simulink model "lab3_simulink"  (R2023b)
settings: Solver=VariableStepAuto  StartTime=0.0  StopTime=150  RelTol=1e-3
values from neighbouring files (symbols this model uses):
  G = tf(num, den, 'IOdelay', Tm)    [lab3.m]
  HR = tf(numHR, denHR, Ts)    [lab3.m]
  HR1 = tf(numHR, denHR1, Ts)    [lab3.m]
settings Model: Creator=Voic  LastModifiedBy=Voic
settings OptimizationCC: ReuseModelBlockBuffer=off

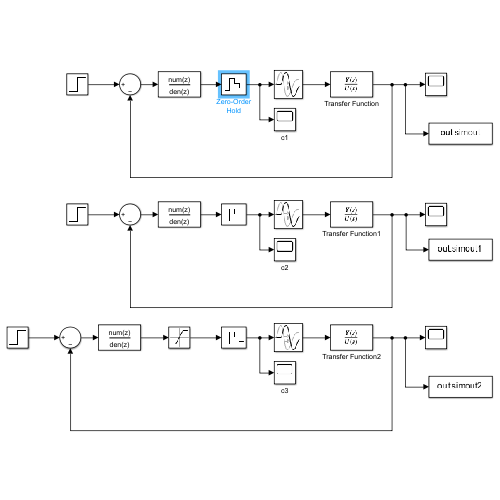
[thumbnail: Simulink's stored preview of the top-level diagram]
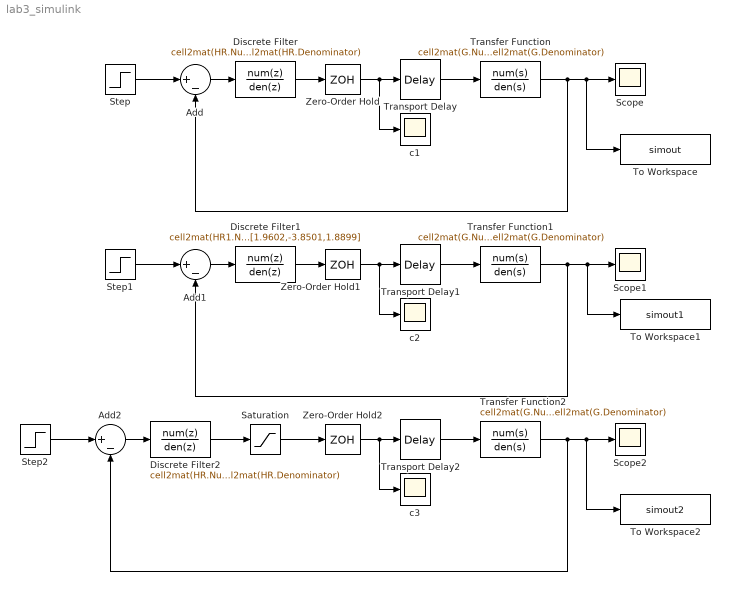
== system lab3_simulink ==
  Add : Sum  Inputs=|+-
  Add1 : Sum  Inputs=|+-
  Add2 : Sum  Inputs=|+-
  Discrete Filter : DiscreteFilter  Numerator=cell2mat(HR.Numerator)  Denominator=cell2mat(HR.Denominator)
  Discrete Filter1 : DiscreteFilter  Numerator=cell2mat(HR1.Numerator)  Denominator=[1.9602,-3.8501,1.8899]
  Discrete Filter2 : DiscreteFilter  Numerator=cell2mat(HR.Numerator)  Denominator=cell2mat(HR.Denominator)
  Saturation : Saturate  UpperLimit=3  LowerLimit=-3
  Scope : Scope
  Scope1 : Scope
  Scope2 : Scope
  Step : Step  SampleTime=0
  Step1 : Step  SampleTime=0
  Step2 : Step  SampleTime=0
  To Workspace : ToWorkspace  VariableName=simout  SaveFormat=Timeseries  SampleTime=-1
  To Workspace1 : ToWorkspace  VariableName=simout1  SaveFormat=Timeseries  SampleTime=-1
  To Workspace2 : ToWorkspace  VariableName=simout2  SaveFormat=Timeseries  SampleTime=-1
  Transfer Function : TransferFcn  Numerator=cell2mat(G.Numerator)  Denominator=cell2mat(G.Denominator)
  Transfer Function1 : TransferFcn  Numerator=cell2mat(G.Numerator)  Denominator=cell2mat(G.Denominator)
  Transfer Function2 : TransferFcn  Numerator=cell2mat(G.Numerator)  Denominator=cell2mat(G.Denominator)
  Transport Delay : TransportDelay  DelayTime=2.5
  Transport Delay1 : TransportDelay  DelayTime=2.5
  Transport Delay2 : TransportDelay  DelayTime=2.5
  Zero-Order Hold : ZeroOrderHold  SampleTime=0.5
  Zero-Order Hold1 : ZeroOrderHold  SampleTime=0.5
  Zero-Order Hold2 : ZeroOrderHold  SampleTime=0.5
  c1 : Scope
  c2 : Scope
  c3 : Scope
  wires:
  Step/1 -> Add/1
  Transfer Function/1 -> Add/2, To Workspace/1, Scope/1
  Add/1 -> Discrete Filter/1
  Discrete Filter/1 -> Zero-Order Hold/1
  Transport Delay/1 -> Transfer Function/1
  Zero-Order Hold/1 -> c1/1, Transport Delay/1
  Discrete Filter1/1 -> Zero-Order Hold1/1
  Add1/1 -> Discrete Filter1/1
  Transfer Function1/1 -> Add1/2, To Workspace1/1, Scope1/1
  Step1/1 -> Add1/1
  Transport Delay1/1 -> Transfer Function1/1
  Zero-Order Hold1/1 -> c2/1, Transport Delay1/1
  Discrete Filter2/1 -> Saturation/1
  Transfer Function2/1 -> Add2/2, To Workspace2/1, Scope2/1
  Add2/1 -> Discrete Filter2/1
  Step2/1 -> Add2/1
  Transport Delay2/1 -> Transfer Function2/1
  Zero-Order Hold2/1 -> c3/1, Transport Delay2/1
  Saturation/1 -> Zero-Order Hold2/1
